simulink model "bpsk_hdl_cosim"  (R2025b)
settings: Solver=FixedStepDiscrete  StartTime=0.0  StopTime=10000/64000  FixedStep=1/64000  RelTol=1e-3
libraries: hdlsllib x1
settings Model: Creator=zizim  LastModifiedBy=zizim
settings OptimizationCC: BlockReduction=off  ConditionallyExecuteInputs=off

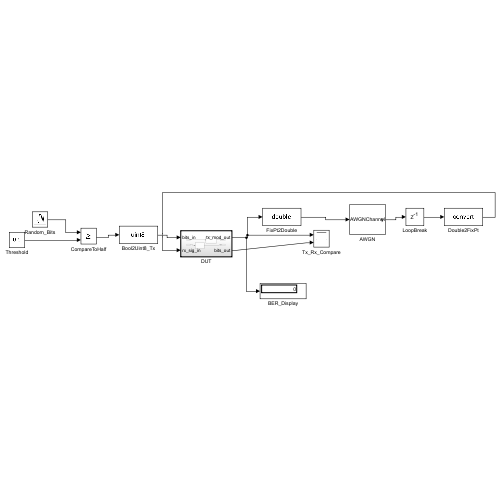
[thumbnail: Simulink's stored preview of the top-level diagram]
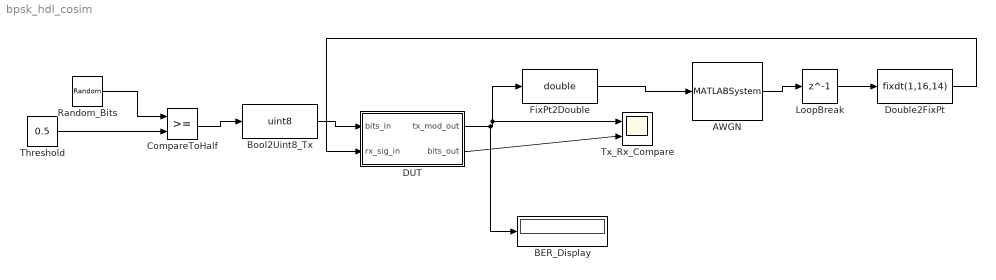
== system bpsk_hdl_cosim ==
  AWGN : MATLABSystem  System=comm.AWGNChannel  NoiseMethod=Signal to noise ratio (Eb/No)  EbNo=10  EsNo=10  SNR=10  BitsPerSymbol=1  SignalPower=1  SamplesPerSymbol=1  VarianceSource=Property  Variance=1  RandomStream=mt19937ar with seed  Seed=67  SimulateUsing=Code generation
      mask Type: comm.AWGNChannel
  BER_Display : Display
  Bool2Uint8_Tx : DataTypeConversion  OutDataTypeStr=uint8
  CompareToHalf : RelationalOperator  OutDataTypeStr=boolean  InputSameDT=off
  DUT : Subsystem  TreatAsAtomicUnit=on
  Double2FixPt : DataTypeConversion  OutDataTypeStr=fixdt(1,16,14)  SaturateOnIntegerOverflow=off  RndMeth=Floor
  FixPt2Double : DataTypeConversion  OutDataTypeStr=double
  LoopBreak : Delay  DelayLength=1
  Random_Bits : RandomNumber  Mean=0.5  Variance=0.25  SampleTime=1/64000
  Threshold : Constant  Value=0.5
  Tx_Rx_Compare : Scope  NumInputPorts=2
  wires:
  Double2FixPt/1 -> DUT/2(rx_sig_in)
  LoopBreak/1 -> Double2FixPt/1
  CompareToHalf/1 -> Bool2Uint8_Tx/1
  Threshold/1 -> CompareToHalf/2
  AWGN/1 -> LoopBreak/1
  DUT/1(tx_mod_out) -> FixPt2Double/1, Tx_Rx_Compare/1, BER_Display/1
  Bool2Uint8_Tx/1 -> DUT/1(bits_in)
  Random_Bits/1 -> CompareToHalf/1
  FixPt2Double/1 -> AWGN/1
  DUT/2(bits_out) -> Tx_Rx_Compare/2

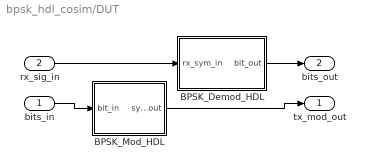
== system bpsk_hdl_cosim/DUT ==
  bits_in : Inport  OutDataTypeStr=uint8
  rx_sig_in : Inport  Port=2
  BPSK_Demod_HDL : Subsystem
  BPSK_Mod_HDL : Subsystem
  tx_mod_out : Outport  VectorParamsAs1DForOutWhenUnconnected=off
  bits_out : Outport  Port=2  VectorParamsAs1DForOutWhenUnconnected=off
  wires:
  rx_sig_in/1 -> BPSK_Demod_HDL/1(rx_sym_in)
  BPSK_Mod_HDL/1(sym_out) -> tx_mod_out/1
  BPSK_Demod_HDL/1(bit_out) -> bits_out/1
  bits_in/1 -> BPSK_Mod_HDL/1(bit_in)

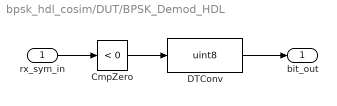
== system bpsk_hdl_cosim/DUT/BPSK_Demod_HDL ==
  rx_sym_in : Inport  OutDataTypeStr=fixdt(1,16,14)
  CmpZero : hdlsllib/Logic and Bit Operations/Compare To Zero  relop=<  OutDataTypeStr=boolean
  DTConv : DataTypeConversion  OutDataTypeStr=uint8
  bit_out : Outport  OutDataTypeStr=uint8  VectorParamsAs1DForOutWhenUnconnected=off
  wires:
  DTConv/1 -> bit_out/1
  CmpZero/1 -> DTConv/1
  rx_sym_in/1 -> CmpZero/1

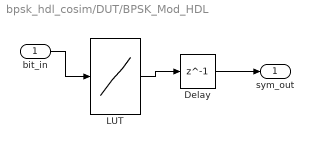
== system bpsk_hdl_cosim/DUT/BPSK_Mod_HDL ==
  bit_in : Inport  OutDataTypeStr=uint8
  Delay : Delay  DelayLength=1
  LUT : Lookup_n-D  NumberOfTableDimensions=1  BreakpointsForDimension1=uint8([0 1])  Table=fi([1; -1], 1, 16, 14)  InterpMethod=Flat  ExtrapMethod=Clip  OutDataTypeStr=fixdt(1,16,14)
  sym_out : Outport  OutDataTypeStr=fixdt(1,16,14)  VectorParamsAs1DForOutWhenUnconnected=off
  wires:
  Delay/1 -> sym_out/1
  LUT/1 -> Delay/1
  bit_in/1 -> LUT/1
